simulink model "PTC_MBDS_StringFind_Sample"  (R2013a)
settings: Solver=FixedStepDiscrete  StartTime=0.0  StopTime=100  FixedStep=0.02  RelTol=1e-3
libraries: simulink_extras x1, PTC_MBDS_LIB x1
settings Model: Creator=uidl7367  LastModifiedBy=sundeep.tuteja
settings DataIOCC: SignalLoggingSaveFormat=ModelDataLogs
settings OptimizationCC: ExpressionDepthLimit=2147483647  InitFltsAndDblsToZero=on
settings DebuggingCC: SaveWithParameterizedLinksMsg=none  SignalResolutionControl=TryResolveAllWithWarning  InheritedTsInSrcMsg=none  MultiTaskDSMMsg=warning  MultiTaskCondExecSysMsg=none  FcnCallInpInsideContextMsg=UseLocalSettings  StrictBusMsg=Warning
settings RTWCC: IncludeERTFirstTime=on
settings GRTTargetCC: TargetFcnLib=ansi_tfl_tmw.mat  CombineOutputUpdateFcns=off  GRTInterface=on

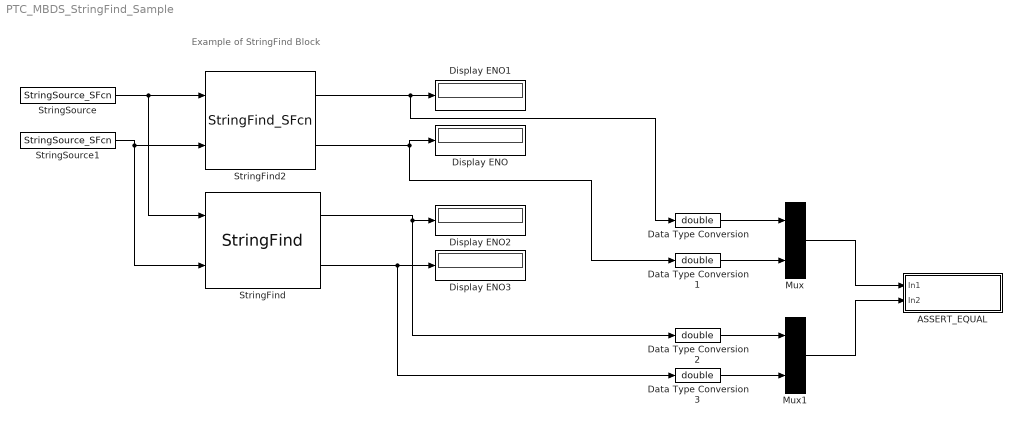
== system PTC_MBDS_StringFind_Sample ==
  note: Example of StringFind Block
  ASSERT_EQUAL : Subsystem
  Data Type Conversion{,1..3} (4 alike) : DataTypeConversion  OutDataTypeStr=double
  Display ENO{,1..3} (4 alike) : Display
  Mux : Mux  Inputs=2
  Mux1 : Mux  Inputs=2
  StringFind : PTC_MBDS_LIB/MBDS Standard Library/Extended Operations/String Operations/StringFind  ENO_Enabled=on  MaxStringLength=PTC_MBDS_MaxStringLength_Fcn  PTC_MBDS_BlockVersion=5.32  PTC_BlockType=PTC_MBDS_StringFind
  StringFind2 : S-Function  InitFcn=|  FunctionName=StringFind_SFcn  Parameters=boolean(ENO_Enabled), uint16(MaxStringLength)  EnableBusSupport=off  mask(StringFind){MBDS_LibraryBlock=on, ENO_Enabled=on, MBDS_BlockVersion=05.40}
      | if(exist('MBDS_BlockCallback', 'file'))
      |    MBDS_BlockCallback('Update', gcb);
      | end
      mask prompts: MBDS_LibraryBlock "MBDS Library Block"; ENO_Enabled "Show ENO port"; MBDS_BlockVersion "Block version:"
      mask help: Searches within the string signal at input port In1 for a substring at input port In2. Result is the first position where In2 is found.
      mask init:
      | MBDS_BlockCallback('Copy', gcb);
      | MaxStringLength = 1 + GetStringLen();
      | maskdisplay = ['disp(''Find'')' 10];
      | maskdisplay = [maskdisplay 'port_label(''input'', 1, ''In1'')' 10];
      | maskdisplay = [maskdisplay 'port_label(''input'', 2, ''In2'')' 10];
      | maskdisplay = [maskdisplay 'port_label(''output'', 1, ''Out'')' 10];
      | if(ENO_Enabled)
      | 	maskdisplay = [maskdisplay 'port_label(''output'', 2, ''ENO'')' 10];
      | end
      | set_param(gcbh, 'maskdisplay', maskdisplay)
      mask Help: eval(['open([workdir(''Library_Dir:''),''\Blockset\Help\'',get_param(gcb,''MaskType''),''.html''])'])
      mask Display:
      | disp('Find')
      | port_label('input', 1, 'In1')
      | port_label('input', 2, 'In2')
      | port_label('output', 1, 'Out')
      | port_label('output', 2, 'ENO')
  StringSource : S-Function  InitFcn=|  FunctionName=StringSource_SFcn  Parameters=uint8(String), uint16(MaxStringLength)  EnableBusSupport=off  mask(StringSource){MBDS_LibraryBlock=on, InputValue=40_character_string_00000000000000000000, MBDS_BlockVersion=05.31}
      | if(exist('MBDS_BlockCallback', 'file'))
      |    MBDS_BlockCallback('Update', gcb);
      | end
      mask prompts: MBDS_LibraryBlock "MBDS Library Block"; InputValue "Constant value:"; MBDS_BlockVersion "Block version:"
      mask help: This block outputs an uint8 array based on the ASCII codes of the string specified by the user.
      mask init:
      | MBDS_BlockCallback('Copy', gcb);
      | MaxStringLength = 1 + GetStringLen();
      | DispString = 'Error';
      | String = InputValue;
      | % Skip if string specifies a numeric expression or starts with '
      | if(isempty(str2num(String)) && String(1) ~= '''')
      |    try
      |       % Try to evaluate project constant 
      |       String = evalin('base', String);
      |    end   
      | end
      | if ~ischar(String) || size(String, 1) > 1
      | 	error('String must be a [1xn] array of type ''char'' with at least one character')
      | else
      |    % Limit to max. string length
      |    String = String(1:min(MaxStringLength, length(String)));
      | 	DispString = InputValue;
      | end
      mask Help: eval(['open([workdir(''Library_Dir:''),''\Blockset\Help\'',get_param(gcb,''MaskType''),''.html''])'])
      mask Display: text(0.05,0.5,DispString,'horizontalAlignment','left')
  StringSource1 : S-Function  InitFcn=|  FunctionName=StringSource_SFcn  Parameters=uint8(String), uint16(MaxStringLength)  EnableBusSupport=off  mask(StringSource){MBDS_LibraryBlock=on, InputValue=ring, MBDS_BlockVersion=05.31}
      | if(exist('MBDS_BlockCallback', 'file'))
      |    MBDS_BlockCallback('Update', gcb);
      | end
      mask prompts: MBDS_LibraryBlock "MBDS Library Block"; InputValue "Constant value:"; MBDS_BlockVersion "Block version:"
      mask help: This block outputs an uint8 array based on the ASCII codes of the string specified by the user.
      mask init: same as PTC_MBDS_StringFind_Sample/StringSource
      mask Help: eval(['open([workdir(''Library_Dir:''),''\Blockset\Help\'',get_param(gcb,''MaskType''),''.html''])'])
      mask Display: text(0.05,0.5,DispString,'horizontalAlignment','left')
  wires:
  StringFind2/1 -> Data Type Conversion/1, Display ENO1/1
  StringFind2/2 -> Display ENO/1, Data Type Conversion1/1
  StringSource/1 -> StringFind/1, StringFind2/1
  StringSource1/1 -> StringFind/2, StringFind2/2
  StringFind/1 -> Data Type Conversion2/1, Display ENO2/1
  StringFind/2 -> Data Type Conversion3/1, Display ENO3/1
  Mux/1 -> ASSERT_EQUAL/1(In1)
  Mux1/1 -> ASSERT_EQUAL/2(In2)
  Data Type Conversion/1 -> Mux/1
  Data Type Conversion1/1 -> Mux/2
  Data Type Conversion2/1 -> Mux1/1
  Data Type Conversion3/1 -> Mux1/2

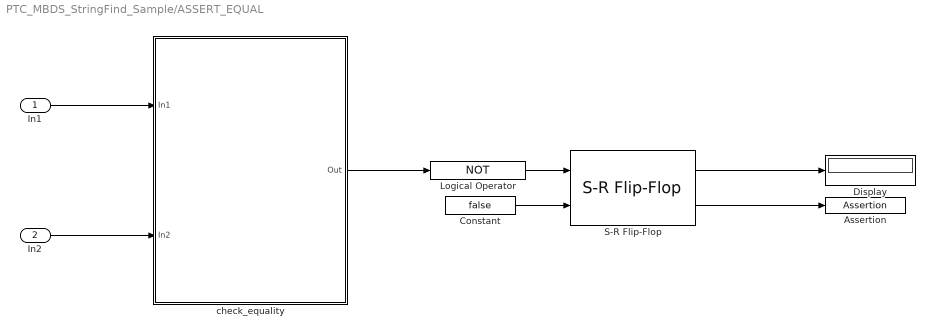
== system PTC_MBDS_StringFind_Sample/ASSERT_EQUAL ==
  In1 : Inport
  In2 : Inport  Port=2
  Assertion : Assertion
  Constant : Constant  Value=false
  Display : Display
  Logical Operator : Logic  Operator=NOT  AllPortsSameDT=off  OutDataTypeStr=boolean
  S-R Flip-Flop : simulink_extras/Flip Flops/S-R Flip-Flop  initial_condition=0
  check_equality : MATLAB Function  TreatAsAtomicUnit=on
  wires:
  S-R Flip-Flop/1 -> Display/1
  check_equality/1(Out) -> Logical Operator/1
  Constant/1 -> S-R Flip-Flop/2
  S-R Flip-Flop/2 -> Assertion/1
  In2/1 -> check_equality/2(In2)
  In1/1 -> check_equality/1(In1)
  Logical Operator/1 -> S-R Flip-Flop/1

== matlab function PTC_MBDS_StringFind_Sample/ASSERT_EQUAL/check_equality ==
  data: In1 input; Out output; In2 input
function Out = check_equality(In1, In2)
%#codegen

Out = isequaln(In1, In2);

end
